simulink model "single_phase_grid_inverter"  (R2022b)
settings: Solver=FixedStepDiscrete  StartTime=0.0  StopTime=1.2  FixedStep=1e-6  RelTol=1e-3
libraries: spsSeriesRLCBranchLib x10, spsCurrentMeasurementLib x7, spsMosfetLib x6, spsVoltageMeasurementLib x6, spsFourierLib x4, spsRMSLib x4, spsIdealSwitchLib x2, spsMeanLib x2, simulink x2, spsDCVoltageSourceLib x1, spspowerguiLib x1, spsControlledVoltageSourceLib x1
settings Model: Creator=XIAO  LastModifiedBy=XIAO
settings SolverCC: AutoInsertRateTranBlk=on
settings DataIOCC: ReturnWorkspaceOutputs=off

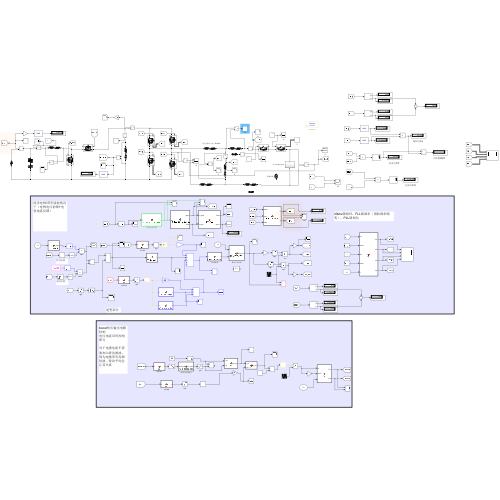
[thumbnail: Simulink's stored preview of the top-level diagram]
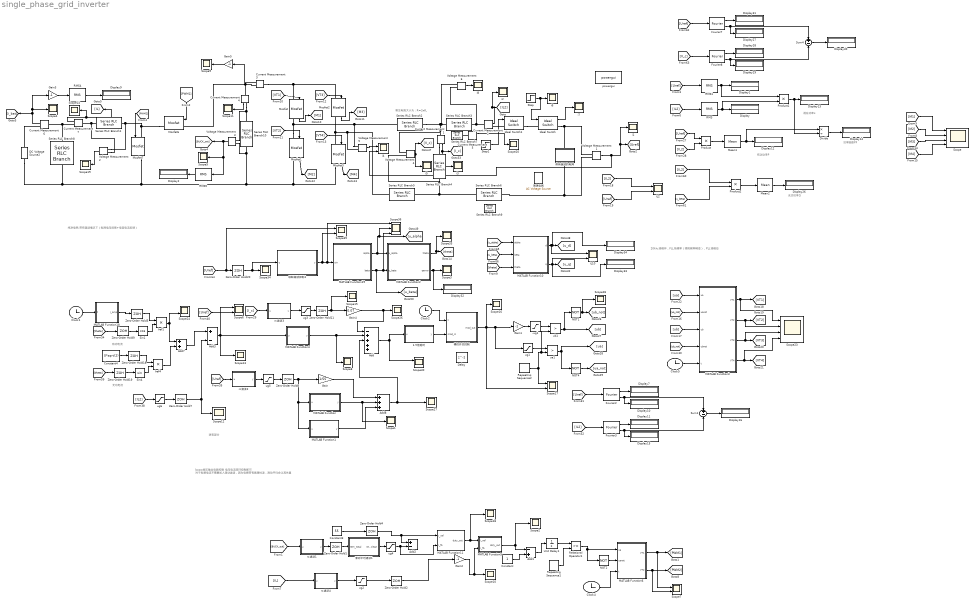
== system single_phase_grid_inverter ==
  note: 视在功率s
  note: 寄生电阻大小为：R=2πfL
  note: 功率因数PF
  note: 无功功率Q
  note: 有功电流
  note: 无功电流
  note: 纯净电网/带有谐波情况下（电网电压前馈+电容电流反馈）
  note: 有功功率P
  note: 逆变部分
  note: 20khz锁相环，FLL锁频率（预防频率畸变），PLL锁相位
  note: boost恒压输出电路控制
      | 电压电流双环控制即可
      |
      | 对于电感电流不需要加入滑动滤波，因为电感带有高频纹波，滑动平均会让其失真
  -ug1 : Saturate  UpperLimit=0.95  LowerLimit=-0.95
  1.5倍延时 : MATLAB Function  TreatAsAtomicUnit=on
  Add : Sum  Inputs=-++++
  Add1 : Sum  Inputs=-+
  Add2 : Sum  Inputs=+-
  Add3 : Sum  Inputs=+-
  Add7 : Sum
  Add8 : Sum  Inputs=+++
  Clock{1..2,4..5} (4 alike) : Clock
  Constant : Constant
  Constant3 : Constant  Value=55
  Constant4 : Constant  Value=0*sqrt(2)
  Current Measurement{1..7} (7 alike) : spsCurrentMeasurementLib/Current Measurement  PhasorSimulation=off  OutputType=Complex  PSBequivalent=0
  DC Voltage Source2 : spsDCVoltageSourceLib/DC Voltage Source  Amplitude=24  Measurements=None
  Delay : Delay  DelayLength=1  SampleTime=5e-5
  Display{,1..2,7,9..16,26..34} (21 alike) : Display
  Divide : Product  Inputs=*/
  Fourier{2..3,7..8} (4 alike) : spsFourierLib/Fourier  Freq=50  n=1  InInit=[0, 0]  Ts=1e-6
  Gain : Gain  Gain=1/55
  Gain{1..3,5} (4 alike) : Gain  Gain=-1
  Gain4 : Gain  Gain=0.07
  Ideal Switch : spsIdealSwitchLib/Ideal Switch  Ron=0.001  Lon=0  IC=0  Rs=1e5  Cs=inf  Measurements=on
  Ideal Switch1 : spsIdealSwitchLib/Ideal Switch  Ron=0.001  Lon=0  IC=0  Rs=1e5  Cs=inf  Measurements=on
  Iref1 : Product
  Iref4 : Product
  MATLAB Function : MATLAB Function  TreatAsAtomicUnit=on
  MATLAB Function1 : MATLAB Function  TreatAsAtomicUnit=on
  MATLAB Function10 : MATLAB Function  TreatAsAtomicUnit=on
  MATLAB Function11 : MATLAB Function  TreatAsAtomicUnit=on
  MATLAB Function18 : MATLAB Function  TreatAsAtomicUnit=on
  MATLAB Function19 : MATLAB Function  TreatAsAtomicUnit=on
  MATLAB Function2 : MATLAB Function  TreatAsAtomicUnit=on
  MATLAB Function3 : MATLAB Function  TreatAsAtomicUnit=on
  MATLAB Function4 : MATLAB Function  TreatAsAtomicUnit=on
  MATLAB Function5 : MATLAB Function  TreatAsAtomicUnit=on
  MATLAB Function6 : MATLAB Function  TreatAsAtomicUnit=on
  Mean1 : spsMeanLib/Mean  Freq=50  Vinit=0  Ts=5e-5
  Mean2 : spsMeanLib/Mean  Freq=50  Vinit=0  Ts=5e-5
  Mosfet{,1..3,6..7} (6 alike) : spsMosfetLib/Mosfet  Ron=0.1  Lon=0  Rd=0.01  Vfd=0  IC=0  Rs=1e5  Cs=inf  Measurements=on
  NOT1 : Logic  Operator=NOT  IconShape=distinctive  AllPortsSameDT=off  OutDataTypeStr=boolean
  NOT2 : Logic  Operator=NOT  IconShape=distinctive  AllPortsSameDT=off  OutDataTypeStr=boolean
  NOT4 : Logic  Operator=NOT  IconShape=distinctive  AllPortsSameDT=off  OutDataTypeStr=boolean
  Product : Product
  Product1 : Product
  Product2 : Product
  RMS : spsRMSLib/RMS  TrueRMS=on  Freq=50  RMSInit=24  Ts=1e-6
  RMS1 : spsRMSLib/RMS  TrueRMS=on  Freq=50  RMSInit=24  Ts=1e-6
  RMS4 : spsRMSLib/RMS  TrueRMS=on  Freq=50  RMSInit=120  Ts=1e-6
  RMS5 : spsRMSLib/RMS  TrueRMS=on  Freq=50  RMSInit=120  Ts=1e-6
  Relational Operator1 : RelationalOperator  OutDataTypeStr=boolean  RndMeth=Simplest  InputSameDT=off
  Repeating Sequence1 : simulink/Sources/Repeating Sequence  rep_seq_t=[0 0.00005 0.0001]  rep_seq_y=[0 1 0]
  Repeating Sequence2 : simulink/Sources/Repeating Sequence  rep_seq_t=[0, 5e-5, 1e-4]  rep_seq_y=[-1, 1, -1]
  Scope : Scope  NumInputPorts=4
  Scope{1..5,8..16,18..20,26..28,33..34} (22 alike) : Scope
  Scope{6..7,17,24,30,35} (6 alike) : Scope  NumInputPorts=2
  Scope23 : Scope  NumInputPorts=4
  Scope36 : Scope  NumInputPorts=3
  Series RLC Branch1 : spsSeriesRLCBranchLib/Series RLC Branch  LConnTagsString=__new0  RConnTagsString=__new0  BranchType=RL  Resistance=0.1  Inductance=2.5e-3  SetiL0=off  InitialCurrent=0  Capacitance=1e-6  Setx0=off  InitialVoltage=0  Measurements=None
  Series RLC Branch10 : spsSeriesRLCBranchLib/Series RLC Branch  LConnTagsString=__new0  RConnTagsString=__new0  BranchType=RC  Resistance=0.01  Inductance=0  SetiL0=off  InitialCurrent=0  Capacitance=1880e-6  Setx0=off  InitialVoltage=0  Measurements=None
  Series RLC Branch2 : spsSeriesRLCBranchLib/Series RLC Branch  LConnTagsString=__new0  RConnTagsString=__new0  BranchType=RL  Resistance=0.1  Inductance=0.0015  SetiL0=off  InitialCurrent=0  Capacitance=220e-6  Setx0=off  InitialVoltage=0  Measurements=None
  Series RLC Branch3 : spsSeriesRLCBranchLib/Series RLC Branch  LConnTagsString=__new0  RConnTagsString=__new0  BranchType=RL  Resistance=0.1  Inductance=0.00012  SetiL0=off  InitialCurrent=0  Capacitance=220e-6  Setx0=off  InitialVoltage=0  Measurements=None
  Series RLC Branch4 : spsSeriesRLCBranchLib/Series RLC Branch  LConnTagsString=__new0  RConnTagsString=__new0  BranchType=RC  Resistance=0.1  Inductance=0  SetiL0=off  InitialCurrent=0  Capacitance=10e-6  Setx0=off  InitialVoltage=0  Measurements=None
  Series RLC Branch5 : spsSeriesRLCBranchLib/Series RLC Branch  LConnTagsString=__new0  RConnTagsString=__new0  BranchType=RL  Resistance=0.1  Inductance=0.0015  SetiL0=off  InitialCurrent=0  Capacitance=220e-6  Setx0=off  InitialVoltage=0  Measurements=None
  Series RLC Branch6 : spsSeriesRLCBranchLib/Series RLC Branch  LConnTagsString=__new0  RConnTagsString=__new0  BranchType=RL  Resistance=0.1  Inductance=0.00012  SetiL0=off  InitialCurrent=0  Capacitance=220e-6  Setx0=off  InitialVoltage=0  Measurements=None
  Series RLC Branch7 : spsSeriesRLCBranchLib/Series RLC Branch  LConnTagsString=__new0  RConnTagsString=__new0  BranchType=RC  Resistance=10  Inductance=0.0000001  SetiL0=off  InitialCurrent=0  Capacitance=1e-7  Setx0=off  InitialVoltage=0  Measurements=None
  Series RLC Branch8 : spsSeriesRLCBranchLib/Series RLC Branch  LConnTagsString=__new0  RConnTagsString=__new0  BranchType=RC  Resistance=0.1  Inductance=1e-3  SetiL0=off  InitialCurrent=0  Capacitance=940e-6  Setx0=off  InitialVoltage=0  Measurements=None
  Series RLC Branch9 : spsSeriesRLCBranchLib/Series RLC Branch  LConnTagsString=__new0  RConnTagsString=__new0  BranchType=RC  Resistance=10  Inductance=0.0000001  SetiL0=off  InitialCurrent=0  Capacitance=1e-7  Setx0=off  InitialVoltage=0  Measurements=None
  Sin1 : Trigonometry  Operator=cos
  Sin4 : Trigonometry
  Step : Step  Time=0.26  SampleTime=1e-6
  Step1 : Step  Before=1  After=0  SampleTime=1e-6
  Sum1 : Sum  Inputs=+-
  Sum4 : Sum  Inputs=+-
  Unit Delay1 : UnitDelay  SampleTime=5e-5  HasFrameUpgradeWarning=on
  Voltage Measurement{1..6} (6 alike) : spsVoltageMeasurementLib/Voltage Measurement  PhasorSimulation=off  OutputType=Complex  PSBequivalent=0
  Zero-Order Hold{1..2,4..5,7..9,11,18..20} (11 alike) : ZeroOrderHold  SampleTime=5e-5
  i{1..3,5..8} (7 alike) : Scope
  i4 : Scope  NumInputPorts=2
  iL10 : Scope  NumInputPorts=2
  iL2 : Scope  NumInputPorts=2
  powergui : spspowerguiLib/powergui  Priority=1  SimulationMode=Discrete  SampleTime=1e-6  frequency=60  Iterations=50  frequencyindice=0  Pbase=100e6  ErrMax=1e-4  UnitsV=kV  UnitsW=MW  buscounter=0  FunctionMessages=off  echomessages=off  EnableUseOfTLC=off  CurrentSourceSwitches=off  DisableSnubberDevices=off  DisableRonSwitches=off  DisableVfSwitches=off  DisplayEquations=off  AutomaticDiscreteSolvers=off  SolverType=Tustin/Backward Euler (TBE)  Interpol=off  ExternalGateDelay=off  methode=off  Ts=100  x0status=blocks  SPID=on  SwTol=0  HookPort=off  NonlinearTolerance=1e-4  nMaxIteration=100  ContinueOnMaxIteration=off  RestoreLinks=warning  ResistiveCurrentMeasurement=off  Frange=[0:2:500]  Ylog=off  Xlog=on  ShowGrid=off  save=off  variable=ZData  structure=0  ZoomFFT=off  StartTime=0.0  cycles=1  DisplayStyle=1  fundamental=60  FreqAxis=off  MaxFrequency=1000  frequencyindicesteady=1  RmsSteady=1  display=off
  rc滤波1 : MATLAB Function  TreatAsAtomicUnit=on
  rc滤波2 : MATLAB Function  TreatAsAtomicUnit=on
  rc滤波3 : MATLAB Function  TreatAsAtomicUnit=on
  rc滤波4 : MATLAB Function  TreatAsAtomicUnit=on
  ua1 : RelationalOperator  Operator=>  OutDataTypeStr=boolean  RndMeth=Simplest  InputSameDT=off
  ub1 : RelationalOperator  Operator=>  OutDataTypeStr=boolean  RndMeth=Simplest  InputSameDT=off
  ug1 : Saturate  UpperLimit=0.95  LowerLimit=-0.95
  ug2 : Saturate  UpperLimit=10  LowerLimit=-10
  ug3 : Saturate  UpperLimit=5  LowerLimit=-5
  ug4 : Saturate  UpperLimit=60  LowerLimit=-60
  ug5 : Saturate  UpperLimit=5  LowerLimit=-5
  ug6 : Saturate  UpperLimit=10  LowerLimit=-10
  带有谐波的电网 : Subsystem
  模仿开关控制 : MATLAB Function  TreatAsAtomicUnit=on
  滑动平均滤波1 : MATLAB Function  TreatAsAtomicUnit=on
  理想电网 : spsACVoltageSourceLib/AC Voltage Source  Amplitude=24*1.414  Phase=0  Frequency=50  SampleTime=0  Measurements=None  BusType=swing  Pref=10e3  Qref=0  Qmin=-inf  Qmax=+inf
  级联谐波抑制4 : MATLAB Function  TreatAsAtomicUnit=on
  wires:
  [theta] -> Zero-Order Hold9/1
  [M2] -> Scope/2
  Fourier2/2 -> Display10/1, Sum1/1
  [VT1] -> Mosfet/1
  NOT1/1 -> Scope28/1, [ub_not]
  ub1/1 -> [ub], NOT1/1
  [M3] -> Scope/3
  Sin1/1 -> Iref1/2
  Fourier3/1 -> Display11/1
  Mean1/1 -> Divide/1, Display12/1
  [VT3] -> Mosfet2/1
  [IL2] -> Product/2
  [Uref] -> Product/1
  Product/1 -> Mean1/1
  [Uref] -> RMS1/1
  [IL2] -> RMS/1
  [VT4] -> Mosfet3/1
  [M1] -> Scope/1
  RMS/1 -> Product1/2, Display/1
  Sum1/1 -> Display16/1
  Add8/1 -> Add/3, Scope27/1
  模仿开关控制/1(mod_out) -> Scope16/1, Gain1/1, ug1/1, Scope17/2
  Iref4/1 -> Add7/2
  Fourier7/1 -> Display31/1
  1.5倍延时/1(y) -> 模仿开关控制/2(mod_in)
  Fourier8/2 -> Sum4/2, Display29/1
  MATLAB Function18/1(I_amp) -> Zero-Order Hold5/1
  Add/1 -> 1.5倍延时/1(u), Scope30/1
  Mean2/1 -> Display26/1
  Repeating Sequence2/1 -> ub1/2, ua1/2, Scope17/1
  [IL2] -> Product2/1
  Fourier8/1 -> Display28/1
  Zero-Order Hold9/1 -> Sin1/1
  Fourier2/1 -> Display7/1
  Gain4/1 -> Scope26/1, Add/1
  Zero-Order Hold7/1 -> Add3/2, Scope12/1
  Clock2/1 -> 模仿开关控制/1(t)
  MATLAB Function4/1(y) -> Add/2, Scope8/1
  [V_c] -> Fourier8/1
  Sum4/1 -> Display30/1
  Fourier7/2 -> Display27/1, Sum4/1
  [Uref] -> Fourier2/1
  Gain1/1 -> -ug1/1
  [Uref] -> Fourier7/1
  -ug1/1 -> ub1/1
  Gain/1 -> Add8/1
  Fourier3/2 -> Sum1/2, Display15/1
  Clock1/1 -> MATLAB Function18/1(t)
  Ideal Switch/1 -> i7/1
  Step/1 -> Ideal Switch/1, i6/1
  [I_c] -> rc滤波3/1(u)
  [theta] -> Zero-Order Hold19/1
  Product1/1 -> Divide/2, Display13/1
  Sin4/1 -> Iref4/2
  Current Measurement2/1 -> [IL2], i2/1
  Add3/1 -> Scope6/1, MATLAB Function4/1(u), Scope13/1
  [IL2] -> Fourier3/1
  Zero-Order Hold18/1 -> Iref4/1
  Product2/1 -> Mean2/1
  Zero-Order Hold19/1 -> Sin4/1
  [Uref] -> iL2/2
  RMS1/1 -> Product1/1, Display1/1
  MATLAB Function/1(y) -> Scope1/1, Add8/2
  Constant4/1 -> Zero-Order Hold18/1
  NOT4/1 -> [ua_not]
  Zero-Order Hold5/1 -> Iref1/1
  Mosfet/1 -> [M1]
  [IL2] -> ug6/1
  ug1/1 -> ua1/1
  Zero-Order Hold8/1 -> MATLAB Function1/1(u), MATLAB Function/1(u), Gain/1
  [Uref] -> rc滤波2/1(u)
  Current Measurement1/1 -> [I_c], i3/1
  Mosfet1/1 -> [M2]
  [u_beta] -> Product2/2
  Voltage Measurement4/1 -> i5/1, [V_c]
  [VT2] -> Mosfet1/1
  Mosfet3/1 -> [M4]
  ua1/1 -> [ua], NOT4/1
  Voltage Measurement1/1 -> i4/2, i1/1, [Uref]
  [M4] -> Scope/4
  [IL2] -> iL2/1
  Divide/1 -> Display14/1
  Add7/1 -> Add3/1
  Iref1/1 -> Add7/1, Scope24/2
  Mosfet2/1 -> [M3]
  [Uref] -> Scope6/2
  Zero-Order Hold2/1 -> Gain2/1
  MATLAB Function11/1(duty_out) -> Scope18/1, MATLAB Function5/1(I_ref)
  Repeating Sequence1/1 -> Relational Operator1/2
  Gain2/1 -> Scope10/1, MATLAB Function5/2(I_fb)
  Zero-Order Hold1/1 -> 滑动平均滤波1/1(IGm_total)
  Unit Delay1/1 -> Relational Operator1/1
  [BUCK_out] -> rc滤波1/1(u)
  Relational Operator1/1 -> NOT2/1, MATLAB Function6/1(ua)
  RMS4/1 -> Display9/1
  Voltage Measurement3/1 -> RMS5/1, Scope5/1, [BUCK_out]
  [PWM1] -> Mosfet6/1
  RMS5/1 -> Display2/1
  Current Measurement6/1 -> [i_bat], Scope4/1, Gain3/1
  [PWM2] -> Mosfet7/1
  Gain3/1 -> RMS4/1
  Current Measurement3/1 -> Gain5/1
  Gain5/1 -> Scope9/1
  Current Measurement4/1 -> Scope11/1
  Current Measurement7/1 -> Scope14/1, [IL]
  MATLAB Function2/2(qerror) -> Scope3/1, Display32/1
  MATLAB Function19/1(alpha) -> Scope36/2, [u_alpha], MATLAB Function2/1(u_alpha)
  MATLAB Function19/2(beta) -> Scope36/3, MATLAB Function2/2(u_beta), [u_beta]
  [u_alpha] -> MATLAB Function10/1(alpha)
  Zero-Order Hold20/1 -> 级联谐波抑制4/1(u), Scope34/1
  MATLAB Function2/1(theta) -> Scope33/1, [theta]
  级联谐波抑制4/1(y) -> Scope35/2, Scope36/1, MATLAB Function19/1(uin)
  [theta] -> MATLAB Function10/3(theta)
  MATLAB Function10/2(q) -> Display33/1, [u_q], iL10/2
  [Uref] -> Scope35/1, Zero-Order Hold20/1
  MATLAB Function10/1(d) -> iL10/1, Display34/1, [u_d]
  [u_beta] -> MATLAB Function10/2(beta)
  Zero-Order Hold11/1 -> Scope15/1, Gain4/1
  Constant3/1 -> Zero-Order Hold4/1
  Zero-Order Hold4/1 -> MATLAB Function11/1(I_ref), Add2/1
  [IL] -> rc滤波4/1(u)
  ug2/1 -> Zero-Order Hold2/1
  MATLAB Function5/1(duty_out) -> Add1/1, Scope2/1
  ug3/1 -> Zero-Order Hold11/1
  ug4/1 -> MATLAB Function11/2(I_fb), Add2/2
  ug5/1 -> Zero-Order Hold8/1
  MATLAB Function1/1(y) -> Add8/3
  Voltage Measurement2/1 -> Scope19/1
  Clock5/1 -> MATLAB Function3/5(t)
  MATLAB Function3/1(VT1) -> Scope23/1, [VT1]
  [ub] -> MATLAB Function3/3(ub)
  MATLAB Function3/2(VT2) -> Scope23/2, [VT2]
  [ua] -> MATLAB Function3/1(ua)
  MATLAB Function3/3(VT3) -> Scope23/3, [VT3]
  MATLAB Function3/4(VT4) -> Scope23/4, [VT4]
  [ub_not] -> MATLAB Function3/4(ubnot)
  [ua_not] -> MATLAB Function3/2(uanot)
  ug6/1 -> Zero-Order Hold7/1
  Step1/1 -> Ideal Switch1/1
  MATLAB Function6/1(VT1) -> [PWM1], Scope7/1
  NOT2/1 -> MATLAB Function6/2(uanot)
  Clock4/1 -> MATLAB Function6/3(t)
  MATLAB Function6/2(VT2) -> [PWM2], Scope7/2
  Constant/1 -> Add1/2
  Add1/1 -> Unit Delay1/1
  Voltage Measurement5/1 -> i4/1
  rc滤波1/1(y) -> Zero-Order Hold1/1
  rc滤波4/1(y) -> ug2/1
  滑动平均滤波1/1(IGm_clean) -> ug4/1
  rc滤波2/1(y) -> ug5/1
  rc滤波3/1(y) -> ug3/1
  Voltage Measurement6/1 -> i8/1
  Current Measurement5/1 -> Scope20/1
  connections:
  Ideal Switch/RConn1 -- Voltage Measurement1/LConn1 -- 带有谐波的电网/RConn1
  Mosfet2/RConn1 -- Voltage Measurement5/LConn2 -- Series RLC Branch5/RConn1 -- Mosfet3/LConn1
  Voltage Measurement3/LConn2 -- Series RLC Branch10/RConn1 -- Mosfet7/RConn1 -- Series RLC Branch8/RConn1 -- DC Voltage Source2/LConn1 -- Mosfet1/RConn1 -- Mosfet3/RConn1
  Mosfet1/LConn1 -- Voltage Measurement5/LConn1 -- Series RLC Branch2/RConn1 -- Mosfet/RConn1
  Series RLC Branch2/LConn1 -- Current Measurement1/LConn1 -- Voltage Measurement4/LConn1 -- Series RLC Branch3/RConn1 -- Voltage Measurement6/LConn1
  Current Measurement2/LConn1 -- Voltage Measurement6/LConn2 -- Series RLC Branch3/LConn1
  Current Measurement1/RConn1 -- Series RLC Branch4/LConn1
  Series RLC Branch8/LConn1 -- Current Measurement7/RConn1 -- Current Measurement6/LConn1
  Mosfet6/RConn1 -- Voltage Measurement2/LConn1 -- Series RLC Branch1/LConn1 -- Mosfet7/LConn1
  Current Measurement3/RConn1 -- Current Measurement4/LConn1 -- Mosfet6/LConn1
  Series RLC Branch1/RConn1 -- Voltage Measurement2/LConn2 -- Current Measurement7/LConn1
  Current Measurement6/RConn1 -- DC Voltage Source2/RConn1
  Series RLC Branch4/RConn1 -- Voltage Measurement4/LConn2 -- Series RLC Branch6/RConn1 -- Series RLC Branch5/LConn1
  Voltage Measurement1/LConn2 -- 带有谐波的电网/LConn1 -- Series RLC Branch6/LConn1
  Mosfet2/LConn1 -- Current Measurement3/LConn1 -- Mosfet/LConn1
  Voltage Measurement3/LConn1 -- Series RLC Branch10/LConn1 -- Current Measurement4/RConn1
  Ideal Switch1/LConn1 -- Current Measurement2/RConn1
  Ideal Switch1/RConn1 -- Ideal Switch/LConn1
  Current Measurement5/LConn1 -- Series RLC Branch7/LConn1

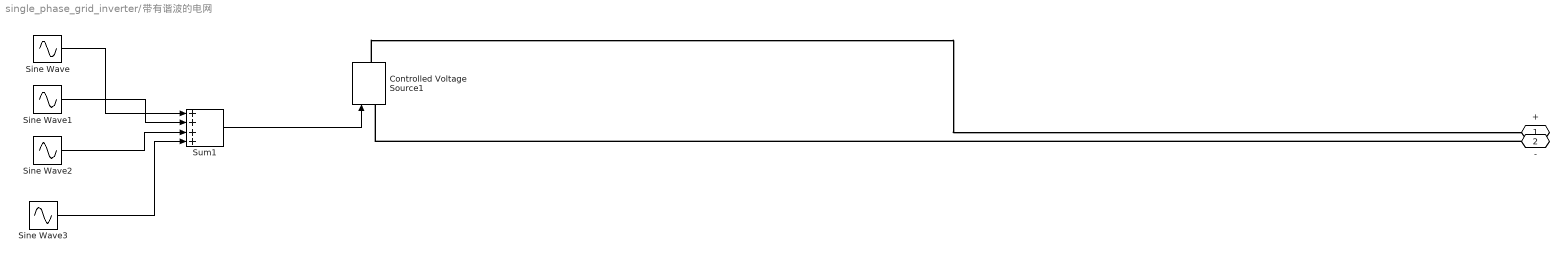
== system single_phase_grid_inverter/带有谐波的电网 ==
  Controlled Voltage Source1 : spsControlledVoltageSourceLib/Controlled Voltage Source  Initialize=off  Source_Type=AC  Amplitude=0  Phase=0  Frequency=0  Measurements=Voltage
  Sine Wave : Sin  Amplitude=32*sqrt(2)  Frequency=100*pi  SampleTime=0
  Sine Wave1 : Sin  Amplitude=0.04*32*sqrt(2)  Frequency=300*pi  SampleTime=0
  Sine Wave2 : Sin  Amplitude=0.03*32*sqrt(2)  Frequency=500*pi  SampleTime=0
  Sine Wave3 : Sin  Amplitude=0.02*32*sqrt(2)  Frequency=700*pi  SampleTime=0
  Sum1 : Sum  Inputs=++++
  + : PMIOPort  Side=Right
  - : PMIOPort  Port=2  Side=Left
  wires:
  Sum1/1 -> Controlled Voltage Source1/1
  Sine Wave1/1 -> Sum1/2
  Sine Wave/1 -> Sum1/1
  Sine Wave3/1 -> Sum1/4
  Sine Wave2/1 -> Sum1/3
  connections:
  -/RConn1 -- Controlled Voltage Source1/LConn1
  Controlled Voltage Source1/RConn1 -- +/RConn1

== matlab function single_phase_grid_inverter/MATLAB Function11 ==
  data: I_ref input; duty_out output; I_fb input
function duty_out = fcn(I_ref, I_fb)
%#codegen
% 同步Boost电流环PI控制器（带钳位抗饱和）
% 适配：20kHz采样、±5A电流传感器、占空比0.1~0.9安全范围
% 输入：
%   I_ref: 电压环输出的电流给定（对应你模型里电压环PI的输出）
%   I_fb: 电流反馈（对应你模型里经过-1增益后的IL信号）
% 输出：
%   duty_out: 最终占空比，直接接你模型里的1/z延迟模块

% 持久化变量：保存积分器状态，每个控制周期保留数值
persistent integral_val;
% 初始化：仅仿真启动的第一个控制周期执行1次
if isempty(integral_val)
    integral_val = 0;
end

% ==================== 1. 控制参数（和你原PI模块参数完全一致，可直接修改）====================
Kp = 0.5;       % 比例增益，和你原设置一致
Ki = 10;         % 积分增益，和你原设置一致
Ts = 5e-5;       % 20kHz控制周期，固定不变
% ==================== 2. 物理极限设置（核心抗饱和阈值）====================
DUTY_MAX = 100;  % 占空比上限，避免上下管直通
DUTY_MIN = -100;  % 占空比下限，杜绝轻载反向电流
I_SAT_LIMIT = 60; % 电流传感器饱和阈值，接近±5A量程提前触发保护

% ==================== 3. 误差计算 ====================
err = I_ref - I_fb;

% ==================== 4. 比例项输出 ====================
prop_out = Kp * err;

% ==================== 5. 核心抗饱和逻辑 ====================
% 5.1 积分项预计算
integral_inc = Ki * Ts * err;
integral_pre = integral_val + integral_inc;
% 5.2 预计算不饱和的PI输出
duty_pre = prop_out + integral_pre;

% 5.3 钳位抗饱和规则：
% 仅当输出在线性区、且电流未达到传感器饱和阈值时，才允许积分累加
% 同时加入反向积分放行规则，避免积分锁死
is_duty_linear = (duty_pre < DUTY_MAX) && (duty_pre > DUTY_MIN);
is_current_unsat = (abs(I_fb) < I_SAT_LIMIT);
is_integral_allow = is_duty_linear && is_current_unsat;
is_reverse_integral = (err > 0 && integral_pre < 0) || (err < 0 && integral_pre > 0);

if is_integral_allow || is_reverse_integral
    integral_val = integral_pre;
end

% ==================== 6. 最终占空比计算 + 硬限幅兜底 ====================
duty_out = prop_out + integral_val;
duty_out = min(max(duty_out, DUTY_MIN), DUTY_MAX);

== matlab function single_phase_grid_inverter/滑动平均滤波1 ==
  data: IGm_total input; IGm_clean output
function IGm_clean = Notch_100Hz_IGm(IGm_total)
    % 【动态窗口滑动平均滤波】专门消除100Hz纹波
    % 采样频率：20kHz，窗口长度：200点（20kHz/100Hz=200）
    % 核心改进：启动前200个点使用动态窗口，完全消除零值误差
    % 输入：IGm_total - 原始带纹波的电流信号
    % 输出：IGm_clean - 滤波后的平滑电流信号
    
    % 持久变量：仅在第一次调用时初始化，后续调用保留值
    persistent buffer   % 环形数据缓冲区
    persistent index    % 缓冲区当前写入索引
    persistent sum_buf  % 窗口内数据累加和（优化计算，避免循环求和）
    persistent sample_count % 已采样总点数（用于动态窗口判断）
    
    N = 200; % 固定窗口长度：100Hz纹波的精确零点
    
    % ====================== 初始化（仅第一次运行执行） ======================
    if isempty(buffer)
        buffer = zeros(1, N);  % 初始化环形缓冲区为全0
        index = 0;             % 索引从0开始
        sum_buf = 0;           % 累加和初始化为0
        sample_count = 0;      % 采样计数初始化为0
    end
    
    % ====================== 更新索引和计数 ======================
    sample_count = sample_count + 1; % 总采样数+1
    index = index + 1;
    if index > N
        index = 1; % 索引越界时回到起点，实现环形结构
    end
    
    % ====================== 核心滤波逻辑 ======================
    if sample_count <= N
        % ---------------------- 阶段1：动态窗口（前200个点） ----------------------
        % 不除以固定的200，而是除以当前已采样的点数
        % 第1个点：输出 = 第1个点 / 1
        % 第10个点：输出 = 前10个点和 / 10
        % ...
        % 第200个点：输出 = 前200个点和 / 200
        sum_buf = sum_buf + IGm_total;
        buffer(index) = IGm_total;
        IGm_clean = sum_buf / sample_count;
    else
        % ---------------------- 阶段2：标准滑动平均（200个点之后） ----------------------
        % 窗口已满，进入标准滑动模式
        % 减去最旧的采样值，加上最新的采样值
        sum_buf = sum_buf - buffer(index) + IGm_total;
        buffer(index) = IGm_total;
        IGm_clean = sum_buf / N;
    end
end

% 
% function IGm_clean = Notch_100Hz_IGm(IGm_total)
%     % 【标准固定窗口滑动平均滤波】专门消除100Hz纹波
%     % 采样频率：20kHz，窗口长度：200点（20kHz/100Hz=200）
%     % 输入：IGm_total - 原始带纹波的电流信号
%     % 输出：IGm_clean - 滤波后的平滑电流信号
%     
%     % 持久变量：仅在第一次调用时初始化，后续调用保留值
%     persistent buffer   % 环形数据缓冲区
%     persistent index    % 缓冲区当前写入索引
%     persistent sum_buf  % 窗口内数据累加和（优化计算，避免循环求和）
%     
%     N = 200; % 固定窗口长度：100Hz纹波的精确零点
%     
%     % ====================== 初始化（仅第一次运行执行） ======================
%     if isempty(buffer)
%         buffer = zeros(1, N);  % 初始化环形缓冲区为全0
%         index = 0;             % 索引从0开始
%         sum_buf = 0;           % 累加和初始化为0
%     end
%     
%     % ====================== 更新环形缓冲区索引 ======================
%     index = index + 1;
%     if index > N
%         index = 1; % 索引越界时回到起点，实现环形结构
%     end
%     
%     % ====================== 核心滤波逻辑（固定窗口） ======================
%     % 减去最旧的采样值，加上最新的采样值
%     sum_buf = sum_buf - buffer(index) + IGm_total;
%     
%     % 将最新的采样值存入缓冲区
%     buffer(index) = IGm_total;
%     
%     % 计算平均值（滤波输出）
%     IGm_clean = sum_buf / N;
% end

== matlab function single_phase_grid_inverter/MATLAB Function18 ==
  data: t input; I_amp output
function I_amp = current_amp_step(t)
% 功能：0.25s前输出0；0.25s~0.6s线性增长到2*sqrt(2)；0.6s后保持最大值不变
% 输入：t - 时间
% 输出：I_amp - 输出电流幅值

persistent I_target t_start t_end;
if isempty(I_target)
    I_target = 2*sqrt(2);  % 目标峰值：2*根号2 ≈2.828
    t_start  = 0.25;       % 线性增长起始时间
    t_end    = 0.6;        % 线性增长结束时间
end

% 分段逻辑
if t < t_start
    % 0 ~ 0.25s：输出0
    I_amp = 0;
elseif t <= t_end
    % 0.25s ~ 0.6s：线性增长计算
    % 公式：当前值 = 目标值 × (当前时间-起始时间)/总增长时间
    I_amp = I_target * (t - t_start) / (t_end - t_start);
else
    % 大于0.6s：保持最大值不变
    I_amp = I_target;
end
end

== matlab function single_phase_grid_inverter/模仿开关控制 ==
  data: t input; mod_out output; mod_in input
function mod_out = gate_mod_signal(t, mod_in)
% 功能：0.25s前输出0，0.25s后输出原调制波mod_in
% 输入 t: 仿真时间 (Clock模块)
% 输入 mod_in: 原始调制波信号
% 输出 mod_out: 带使能的调制波信号

t_start = 0.25; % 合闸时间

if t < t_start
    mod_out = 0;          % 合闸前强制输出0
else
    mod_out = mod_in;      % 合闸后输出原调制波
end
end

== matlab function single_phase_grid_inverter/MATLAB Function10 ==
  data: alpha input; d output; beta input; theta input; q output
function [d, q] = Park_Transform(alpha, beta, theta)
% Park变换模块（直接输入SOGI-FLL的theta，无内部积分）
% 输入：
%   alpha - α轴分量（SOGI-FLL的U_prime）
%   beta  - β轴分量（SOGI-FLL的deltaU_prime）
%   theta - 瞬时相位（SOGI-FLL直接输出的theta）
% 输出：
%   d         - d轴（直轴）分量
%   q         - q轴（交轴）分量
%   cos_theta - 相位θ的余弦值（新增输出）
%   sin_theta - 相位θ的正弦值（新增输出）

%% 核心计算
cos_theta = cos(theta);  % 相位θ的余弦值
sin_theta = sin(theta);  % 相位θ的正弦值


% 修正后的 Park 变换公式（d轴对齐同相分量 beta）
d =  alpha * cos_theta + beta * sin_theta;
q = -alpha * sin_theta + beta * cos_theta;
end

== matlab function single_phase_grid_inverter/MATLAB Function1 ==
  data: u input; y output
function y = GridVoltageFeedforward_Deriv_Module(u)
%#codegen
% 电网电压全前馈二阶微分模块
% 新增：频率预畸变（Frequency Prewarping），修正双线性变换的频率畸变
% 输入u：电网电压采样值 vg
% 输出y：模块输出信号

%% ===================== 1. 系统参数定义 =====================
L1 = 1.5e-3;         % 逆变侧电感，H
C = 10e-6;           % 滤波电容，F
k_pwm = 55;          % PWM桥臂增益
Ts = 1/20000;        % 采样周期，s（20kHz）
f_cutoff = 1150;     % 二阶低通截止频率，Hz（数字域目标频率）
zeta = 0.707;        % 阻尼系数（Butterworth）

%% ===================== 2. 频率预畸变（核心新增） =====================
% 数字域目标角频率
omega_d = 2 * pi * f_cutoff;
% 频率预畸变公式：omega_prewarp = (2/Ts) * tan(omega_d * Ts / 2)
% 目的：让双线性变换后的数字滤波器截止频率精确等于目标f_cutoff
omega_s = (2 / Ts) * tan(omega_d * Ts / 2);

%% ===================== 3. 双线性变换系数计算（使用预畸变后的omega_s） =====================
a = 2 / Ts;  % 双线性变换核心系数
K = (L1 * C) / k_pwm;  % 模块基础比例系数

% 分子系数
num2 = K * (omega_s^2) * (a^2);
num1 = -2 * num2;
num0 = num2;

% 分母系数
den2 = a^2 + 2 * zeta * omega_s * a + omega_s^2;
den1 = -2 * a^2 + 2 * omega_s^2;
den0 = a^2 - 2 * zeta * omega_s * a + omega_s^2;

%% ===================== 4. 状态变量初始化 =====================
persistent u_prev1 u_prev2 y_prev1 y_prev2;
if isempty(u_prev1)
    u_prev1 = 0; % u(k-1)
    u_prev2 = 0; % u(k-2)
    y_prev1 = 0; % y(k-1)
    y_prev2 = 0; % y(k-2)
end

%% ===================== 5. 差分方程实现 =====================
num_part = num2 * u + num1 * u_prev1 + num0 * u_prev2;
den_part = den1 * y_prev1 + den0 * y_prev2;
y = (num_part - den_part) / den2;

%% ===================== 6. 更新状态变量 =====================
u_prev2 = u_prev1;
u_prev1 = u;
y_prev2 = y_prev1;
y_prev1 = y;

end

== matlab function single_phase_grid_inverter/MATLAB Function19 ==
  settings: updateMethod=DISCRETE
  data: uin input; alpha output; beta output
% function [alpha, beta] = SOGI_FLL_20kHz(uin)
% % 严格对应你的 m 文件：20kHz 双线性 PI-FLL
% % 输入：uin   单相电压
% % 输出：alpha 同相输出 uα = x2
% %      beta  正交输出 uβ = omega0*x3
% 
% %% 固定参数（和你的m文件完全一致）
% dt = 5e-5;
% K  = 1.414;
% K1 = 0.25;
% gamma_p =30;
% gamma_i =500;
% w_max = 2*pi*60;
% w_min = 2*pi*40;
% 
% %% 状态持久化
% persistent x1_prev x2_prev x3_prev omega0_prev U_prev integral_f first_run;
% if isempty(first_run)
%     x1_prev = 0;
%     x2_prev = 0;
%     x3_prev = 0;
%     omega0_prev = 2*pi*50;
%     U_prev = uin;
%     integral_f = 0;
%     first_run = false;
% end
% 
% %% 1. 当前输入
% U_curr = uin;
% omega0_prev_local = omega0_prev;
% 
% %% 2. 频率预畸变
% omega_pre = (2/dt) * tan(omega0_prev_local * dt / 2);
% 
% %% 3. 状态矩阵 A, B
% A_mat = [
%     -K1*omega_pre, -K1*omega_pre, 0;
%     -K*omega_pre,  -K*omega_pre,  -omega_pre^2;
%     0,              1,              0
% ];
% B_mat = [
%     K1*omega_pre;
%     K*omega_pre;
%     0
% ];
% 
% %% 4. 双线性变换
% I_mat = eye(3);
% M1 = I_mat - (dt/2)*A_mat;
% M2 = I_mat + (dt/2)*A_mat;
% U_avg = U_curr + U_prev;
% 
% x_prev_vec = [x1_prev; x2_prev; x3_prev];
% x_curr_vec = M1 \ (M2 * x_prev_vec + (dt/2)*B_mat * U_avg);
% 
% x1_curr = x_curr_vec(1);
% x2_curr = x_curr_vec(2);
% x3_curr = x_curr_vec(3);
% 
% %% 5. PI-FLL 频率环
% deltaU = U_curr - x1_curr - x2_curr;
% deltaU_prime_val = omega0_prev_local * x3_curr;
% epsilon_f = deltaU * deltaU_prime_val;
% 
% integral_f = integral_f + epsilon_f * dt;
% domega0dt = -gamma_p * epsilon_f - gamma_i * integral_f;
% omega0_curr = omega0_prev_local + dt * domega0dt;
% 
% % 频率限幅
% omega0_curr = max(min(omega0_curr, w_max), w_min);
% 
% %% 6. 输出 alpha beta
% alpha = x2_curr;
% beta  = omega0_curr * x3_curr;
% 
% %% 7. 更新状态
% x1_prev = x1_curr;
% x2_prev = x2_curr;
% x3_prev = x3_curr;
% omega0_prev = omega0_curr;
% U_prev = U_curr;
% 
% end

function [alpha, beta] = SOGI_FLL_20kHz_Optimized(uin)
% 优化版 SOGI-FLL (针对嵌入式提速)
% 输入：uin - 单相电压采样
% 输出：alpha - 同相分量, beta - 正交分量

%% 固定参数
dt = 5e-5;           % 50us
h  = dt / 2;         % 中间步长
K  = 1.41421356;     % sqrt(2)
K1 = 0.25;
gamma_p = 30;
gamma_i = 500;
w_max = 2 * pi * 60;
w_min = 2 * pi * 40;

%% 状态持久化
persistent x1_prev x2_prev x3_prev omega0_prev U_prev integral_f first_run;
if isempty(first_run)
    x1_prev = 0; x2_prev = 0; x3_prev = 0;
    omega0_prev = 2 * pi * 50;
    U_prev = uin;
    integral_f = 0;
    first_run = false;
end

%% 1. 频率近似 (提速核心 1)
% 原逻辑：omega_pre = (2/dt) * tan(omega0_prev * dt / 2)
% 近似逻辑：当 dt 很小时，tan(x) ≈ x，则 omega_pre ≈ omega0_prev
% 20kHz下，50Hz对应的角度约为 0.0078 rad，近似误差极小
omega_pre = omega0_prev; 
U_avg = uin + U_prev;

%% 2. 预计算常数与中间变量
w_h = omega_pre * h;
wp_sq_h = omega_pre * omega_pre * h;
h_K1w = h * K1 * omega_pre;
h_Kw  = h * K * omega_pre;

% 展开 M2 矩阵与向量乘法: R = M2 * x_prev + h * B * U_avg
% M2 = [1-hK1w, -hK1w, 0; -hKw, 1-hKw, -h*w^2; 0, h, 1]
r1 = (1 - h_K1w)*x1_prev - h_K1w*x2_prev + h_K1w*U_avg;
r2 = -h_Kw*x1_prev + (1 - h_Kw)*x2_prev - wp_sq_h*x3_prev + h_Kw*U_avg;
r3 = h*x2_prev + x3_prev;

%% 3. 代数解析解 (提速核心 2: 消除矩阵求逆)
% 求解 M1 * x_curr = R
% M1 矩阵元素：
% m11 = 1+hK1w; m12 = hK1w; 
% m21 = hKw;    m22 = 1+hKw;  m23 = h*w^2;
% m31 = 0;      m32 = -h;     m33 = 1;

% 利用稀疏性手动降元求解 2x2 方程组
% 步骤 A: x3 = r3 + h*x2
% 步骤 B: 代入第二行消去 x3
a = 1 + h_K1w;
b = h_K1w;
c = h_Kw;
d = 1 + h_Kw + h * wp_sq_h; % 合并项：m22 - m23*(-h)
e = r1;
f = r2 - wp_sq_h * r3;      % 合并项：r2 - m23*r3

% 克莱姆法则求解
det_inv = 1 / (a * d - b * c);
x1_curr = (e * d - b * f) * det_inv;
x2_curr = (a * f - c * e) * det_inv;
x3_curr = r3 + h * x2_curr;

%% 4. FLL 频率环 (保持原逻辑)
deltaU = uin - x1_curr - x2_curr;
epsilon_f = deltaU * (omega_pre * x3_curr);
integral_f = integral_f + epsilon_f * dt;
domega0dt = -gamma_p * epsilon_f - gamma_i * integral_f;
omega0_curr = omega_pre + dt * domega0dt;

% 频率限幅
if omega0_curr > w_max, omega0_curr = w_max; end
if omega0_curr < w_min, omega0_curr = w_min; end

%% 5. 输出与状态更新
alpha = x2_curr;
beta  = omega0_curr * x3_curr;

x1_prev = x1_curr;
x2_prev = x2_curr;
x3_prev = x3_curr;
omega0_prev = omega0_curr;
U_prev = uin;

end

== matlab function single_phase_grid_inverter/MATLAB Function2 ==
  data: u_alpha input; theta output; u_beta input; qerror output
function [theta, qerror] = SRF_PLL(u_alpha, u_beta)
% 同步旋转坐标系锁相环 SRF-PLL
% 【已修改为：纯自适应频率版本 → 和你主循环PLL完全一致】
% 输入：u_alpha, u_beta
% 输出：theta 锁相相位, qerror q分量（趋近0）

    %% ===================== 1. 固定参数 =====================
    Ts = 5e-5;               % 20kHz 采样步长（必须匹配）
    
    % PI参数（和你主循环一致）
    kp_pll = 200;
    ki_pll = 7000;

    %% ===================== 2. 持久变量 =====================
    persistent theta_prev
    persistent integral_pll
    
    if isempty(theta_prev)
        theta_prev = 0;
        integral_pll = 0;
    end

    %% ===================== 3. Park 变换 =====================
    cos_theta = cos(theta_prev);
    sin_theta = sin(theta_prev);
    
    u_d =  u_alpha * cos_theta + u_beta * sin_theta;
    u_q = -u_alpha * sin_theta + u_beta * cos_theta;
    
    qerror = u_q;  % q分量（锁相成功→0）

    %% ===================== 4. PI控制器（我的版本：直接输出ω） =====================
    integral_pll = integral_pll + qerror * Ts;          % 积分
    omega_pll    = kp_pll * qerror + ki_pll * integral_pll; % 直接输出角频率

    %% ===================== 5. 积分生成相位 =====================
    theta = theta_prev + omega_pll * Ts;

    %% ===================== 6. 相位归一化（±π） =====================
    if theta > pi
        theta = theta - 2*pi;
    elseif theta < -pi
        theta = theta + 2*pi;
    end

    %% ===================== 7. 更新状态 =====================
    theta_prev = theta;
end

== matlab function single_phase_grid_inverter/级联谐波抑制4 ==
  data: u input; y output
function y = Cascade_Notch_Filter(u)
% 级联陷波滤波器：滤除3/5/7次固定频率谐波（150/250/350Hz）
% 输入u：待滤波的标量信号
% 输出y：滤波后的标量信号
% 适配：20kHz采样率（Ts=5e-5），和你的控制环完全对齐

    persistent x3_1 x3_2 x5_1 x5_2 x7_1 x7_2 first_run
    persistent b3_0 b3_1 b3_2 a3_1 a3_2
    persistent b5_0 b5_1 b5_2 a5_1 a5_2
    persistent b7_0 b7_1 b7_2 a7_1 a7_2

    %% ===================== 1. 初始化：仅首次运行 =====================
    if isempty(first_run)
        % --- 固定参数 ---
        Fs = 2e4;          % 采样频率 20kHz
        Ts = 1/Fs;            % 采样周期 5e-5s
        wc = 10;              % 截止角频率 25 rad/s
        
        % 目标谐波频率
        w3 = 2*pi*150;  % 3次谐波 150Hz
        w5 = 2*pi*250;  % 5次谐波 250Hz
        w7 = 2*pi*350;  % 7次谐波 350Hz

        % --- Tustin变换预计算系数 ---
        k = 2/Ts;
        k2 = k*k;

        % --- 3次滤波器系数 ---
        [b3_0, b3_1, b3_2, a3_1, a3_2] = calc_coeff(w3, wc, k, k2);
        % --- 5次滤波器系数 ---
        [b5_0, b5_1, b5_2, a5_1, a5_2] = calc_coeff(w5, wc, k, k2);
        % --- 7次滤波器系数 ---
        [b7_0, b7_1, b7_2, a7_1, a7_2] = calc_coeff(w7, wc, k, k2);

        % --- 显式初始化状态变量为标量 ---
        x3_1 = 0; x3_2 = 0;
        x5_1 = 0; x5_2 = 0;
        x7_1 = 0; x7_2 = 0;
        
        first_run = 1;
    end

    %% ===================== 2. 级联滤波计算（显式差分方程） =====================
    % --- 第1级：3次谐波滤波 ---
    y3 = b3_0*u + x3_1;
    x3_1_next = b3_1*u - a3_1*y3 + x3_2;
    x3_2_next = b3_2*u - a3_2*y3;
    
    % --- 第2级：5次谐波滤波 ---
    y5 = b5_0*y3 + x5_1;
    x5_1_next = b5_1*y3 - a5_1*y5 + x5_2;
    x5_2_next = b5_2*y3 - a5_2*y5;
    
    % --- 第3级：7次谐波滤波 ---
    y7 = b7_0*y5 + x7_1;
    x7_1_next = b7_1*y5 - a7_1*y7 + x7_2;
    x7_2_next = b7_2*y5 - a7_2*y7;
    
    % --- 更新状态变量 ---
    x3_1 = x3_1_next; x3_2 = x3_2_next;
    x5_1 = x5_1_next; x5_2 = x5_2_next;
    x7_1 = x7_1_next; x7_2 = x7_2_next;
    
    % --- 最终输出 ---
    y = y7;

end

%% ===================== 局部函数：预计算滤波器系数 =====================
function [b0, b1, b2, a1, a2] = calc_coeff(wn, wc, k, k2)
    % 连续域：G(s) = (s^2 + wn^2) / (s^2 + 2*wc*s + wn^2)
    % Tustin离散化：s = k*(z-1)/(z+1)
    
    % 连续域系数
    num_b0 = 1; num_b1 = 0; num_b2 = wn^2;
    den_a0 = 1; den_a1 = 2*wc; den_a2 = wn^2;
    
    % 离散化计算
    B0 = num_b0*k2 + num_b1*k + num_b2;
    B1 = 2*num_b2 - 2*num_b0*k2;
    B2 = num_b0*k2 - num_b1*k + num_b2;
    
    A0 = den_a0*k2 + den_a1*k + den_a2;
    A1 = 2*den_a2 - 2*den_a0*k2;
    A2 = den_a0*k2 - den_a1*k + den_a2;
    
    % 归一化（a0=1）
    b0 = B0 / A0;
    b1 = B1 / A0;
    b2 = B2 / A0;
    a1 = A1 / A0;
    a2 = A2 / A0;
end

== matlab function single_phase_grid_inverter/MATLAB Function ==
  data: u input; y output
function y = CapCurrentDamping(u)
%#codegen
% 电容电流反馈有源阻尼环节
% 离散化方法：双线性变换法（Tustin），fs=20kHz
% 输入u：电容电压采样值
% 输出y：有源阻尼反馈信号

%% 固定参数（和你的系统匹配）
persistent u_prev  % 上一拍的输入值 u(k-1)
persistent y_prev  % 上一拍的输出值 y(k-1)
C = 10e-6;          % 滤波电容，F
Hi1 = 0.07;          % 反馈系数
Ts = 1/20000;        % 采样周期，s

%% 初始化状态变量
if isempty(u_prev)
    u_prev = 0;
    y_prev = 0;
end

%% 双线性变换法（Tustin）实现微分
% 连续域：G(s) = C*Hi1 * s
% 双线性变换：s = (2/Ts) * (z-1)/(z+1)
% 差分方程：y(k) = -y(k-1) + (2*C*Hi1/Ts) * (u(k) - u(k-1))
K_tustin = (2 * C * Hi1) / Ts;
y = -y_prev + K_tustin * (u - u_prev);

%% 更新状态变量
u_prev = u;
y_prev = y;
end



% function y = CapCurrentDamping_Improved(u)
% %#codegen
% % 电容电流反馈有源阻尼环节（改进版：微分 + 1kHz一阶低通）
% % 特点：绝对稳定，抑制开关噪声，和STM32 C代码逐行对应
% % 离散化方法：双线性变换法（Tustin）+ 频率预畸变，fs=20kHz
% % 输入u：电容电压采样值
% % 输出y：有源阻尼反馈信号
% 
% %% 持久化变量（保存状态和预计算系数）
% persistent u_prev  % 上一拍的输入值 u(k-1)
% persistent y_prev  % 上一拍的输出值 y(k-1)
% persistent b0 b1 a1 % 预计算的离散化系数
% 
% %% 固定参数（和你的系统匹配）
% C = 10e-6;          % 滤波电容，F
% Hi1 = 0.07;          % 反馈系数
% Ts = 1/20000;        % 采样周期，s
% f_cutoff = 1000;     % 【关键】低通截止频率 1kHz
% 
% %% 初始化：仅在第一次运行时执行
% if isempty(u_prev)
%     u_prev = 0;
%     y_prev = 0;
%     
%     % 1. 计算截止角频率
%     omega_c = 2.0 * pi * f_cutoff;
%     
%     % 2. 频率预畸变：让数字截止频率精准对应模拟截止频率
%     omega_s = (2.0 / Ts) * tan(omega_c * Ts / 2.0);
%     
%     % 3. 预计算差分方程系数 (和C代码完全一致)
%     a0 = 2.0 + omega_s * Ts;
%     
%     b0 = (2.0 * C * Hi1 * omega_s) / a0;
%     b1 = -b0;
%     a1 = (omega_s * Ts - 2.0) / a0;
% end
% 
% %% 核心差分方程（每一拍运行）
% % 公式：y(k) = b0*u(k) + b1*u(k-1) - a1*y(k-1)
% y = b0 * u + b1 * u_prev - a1 * y_prev;
% 
% 
% 
% %% 更新状态变量
% u_prev = u;
% y_prev = y;
% 
% end

== matlab function single_phase_grid_inverter/MATLAB Function6 ==
  data: ua input; VT1 output; uanot input; t input; VT2 output
function [VT1, VT2] = fcn(ua, uanot, t)
% 分段 PWM 输出控制
% t < 0.25s       → 全 0
% 0.25s ≤ t < 1s  → 正常输出
% t ≥ 1s          → 再次全 0

if t < 0.9
    VT1 = ua;
    VT2 = uanot;
else
    VT1 = false;
    VT2 = false;
end
   
end

== matlab function single_phase_grid_inverter/MATLAB Function5 ==
  data: I_ref input; duty_out output; I_fb input
function duty_out = fcn(I_ref, I_fb)
%#codegen
% 同步Boost电流环PI控制器（带钳位抗饱和）
% 适配：20kHz采样、±5A电流传感器、占空比0.1~0.9安全范围
% 输入：
%   I_ref: 电压环输出的电流给定（对应你模型里电压环PI的输出）
%   I_fb: 电流反馈（对应你模型里经过-1增益后的IL信号）
% 输出：
%   duty_out: 最终占空比，直接接你模型里的1/z延迟模块

% 持久化变量：保存积分器状态，每个控制周期保留数值
persistent integral_val;
% 初始化：仅仿真启动的第一个控制周期执行1次
if isempty(integral_val)
    integral_val = 0;
end

% ==================== 1. 控制参数（和你原PI模块参数完全一致，可直接修改）====================
Kp = 0.05;       % 比例增益，和你原设置一致
Ki = 10;         % 积分增益，和你原设置一致
Ts = 5e-5;       % 20kHz控制周期，固定不变
% ==================== 2. 物理极限设置（核心抗饱和阈值）====================
DUTY_MAX = 0.85;  % 占空比上限，避免上下管直通
DUTY_MIN = 0.15;  % 占空比下限，杜绝轻载反向电流
I_SAT_LIMIT = 4.5; % 电流传感器饱和阈值，接近±5A量程提前触发保护

% ==================== 3. 误差计算 ====================
err = I_ref - I_fb;

% ==================== 4. 比例项输出 ====================
prop_out = Kp * err;

% ==================== 5. 核心抗饱和逻辑 ====================
% 5.1 积分项预计算
integral_inc = Ki * Ts * err;
integral_pre = integral_val + integral_inc;
% 5.2 预计算不饱和的PI输出
duty_pre = prop_out + integral_pre;

% 5.3 钳位抗饱和规则：
% 仅当输出在线性区、且电流未达到传感器饱和阈值时，才允许积分累加
% 同时加入反向积分放行规则，避免积分锁死
is_duty_linear = (duty_pre < DUTY_MAX) && (duty_pre > DUTY_MIN);
is_current_unsat = (abs(I_fb) < I_SAT_LIMIT);
is_integral_allow = is_duty_linear && is_current_unsat;
is_reverse_integral = (err > 0 && integral_pre < 0) || (err < 0 && integral_pre > 0);

if is_integral_allow || is_reverse_integral
    integral_val = integral_pre;
end

% ==================== 6. 最终占空比计算 + 硬限幅兜底 ====================
duty_out = prop_out + integral_val;
duty_out = min(max(duty_out, DUTY_MIN), DUTY_MAX);

== matlab function single_phase_grid_inverter/rc滤波1 ==
  data: u input; y output
function y = fcn(u)
% 一阶RC低通滤波（数字等效实现）
% 适配：仿真步长 Ts=1e-6s（Fs=1MHz），截止频率 fc=4.7kHz
% 输入：u - 原始信号
% 输出：y - RC滤波后的信号

% persistent 变量保存上一时刻的输出（RC滤波的状态）
persistent y_prev;

% ---------------- 固定参数（已按你的需求预计算） ----------------
fc = 4700;   % 截止频率：4.7kHz
Ts = 1e-6;   % 仿真步长：1us（1e-6s）
tau = 1/(2*pi*fc); % RC时间常数 τ=RC=1/(2πfc)
alpha = exp(-Ts/tau); % 滤波系数（RC离散化核心）
% ----------------------------------------------------------------

% 初始化状态（仅第一次调用时执行，默认初始输出为0）
if isempty(y_prev)
    y_prev = 0;
end

% 一阶RC低通的离散差分方程（和真实RC电路特性完全等效）
y = alpha * y_prev + (1 - alpha) * u;

% 更新状态，为下一个仿真步准备
y_prev = y;

end

== matlab function single_phase_grid_inverter/rc滤波2 ==
  data: u input; y output
function y = fcn(u)
% 一阶RC低通滤波（数字等效实现）
% 适配：仿真步长 Ts=1e-6s（Fs=1MHz），截止频率 fc=4.7kHz
% 输入：u - 原始信号
% 输出：y - RC滤波后的信号

% persistent 变量保存上一时刻的输出（RC滤波的状态）
persistent y_prev;

% ---------------- 固定参数（已按你的需求预计算） ----------------
fc = 4700;   % 截止频率：4.7kHz
Ts = 1e-6;   % 仿真步长：1us（1e-6s）
tau = 1/(2*pi*fc); % RC时间常数 τ=RC=1/(2πfc)
alpha = exp(-Ts/tau); % 滤波系数（RC离散化核心）
% ----------------------------------------------------------------

% 初始化状态（仅第一次调用时执行，默认初始输出为0）
if isempty(y_prev)
    y_prev = 0;
end

% 一阶RC低通的离散差分方程（和真实RC电路特性完全等效）
y = alpha * y_prev + (1 - alpha) * u;

% 更新状态，为下一个仿真步准备
y_prev = y;

end

== matlab function single_phase_grid_inverter/1.5倍延时 ==
  data: u input; y output
function y = SecondOrderPadeDelay_1p5Ts(u)
% 二阶Padé逼近1.5Ts延迟模块（直接从闭环仿真提取，已验证直流增益=1）
% 输入：u - 待延迟的信号（如PR控制器输出）
% 输出：y - 延迟后的信号
% 适配：与你的闭环仿真参数100%匹配，直流增益严格等于1

persistent u_prev1 u_prev2 y_prev1 y_prev2 first_run

%% 初始化：仅首次运行
if isempty(first_run)
    % 初始化状态变量（二阶需要2个历史输入+2个历史输出）
    u_prev1 = 0;
    u_prev2 = 0;
    y_prev1 = 0;
    y_prev2 = 0;
    
    first_run = true;
end

%% 【核心】直接从闭环仿真提取的系数（已验证直流增益=1）
b0 = 0.076923076923077;
b1 = 0.153846153846154;
b2 = 1.000000000000000;
a1 = -0.153846153846154;
a2 = -0.076923076923077;

%% 二阶离散差分方程计算延迟输出
y = b0*u + b1*u_prev1 + b2*u_prev2 ...
    + a1*y_prev1 + a2*y_prev2;

%% 更新状态变量（供下一时刻使用）
u_prev2 = u_prev1;
u_prev1 = u;
y_prev2 = y_prev1;
y_prev1 = y;
end

== matlab function single_phase_grid_inverter/rc滤波3 ==
  data: u input; y output
function y = fcn(u)
% 一阶RC低通滤波（数字等效实现）
% 适配：仿真步长 Ts=1e-6s（Fs=1MHz），截止频率 fc=4.7kHz
% 输入：u - 原始信号
% 输出：y - RC滤波后的信号

% persistent 变量保存上一时刻的输出（RC滤波的状态）
persistent y_prev;

% ---------------- 固定参数（已按你的需求预计算） ----------------
fc = 4700;   % 截止频率：4.7kHz
Ts = 1e-6;   % 仿真步长：1us（1e-6s）
tau = 1/(2*pi*fc); % RC时间常数 τ=RC=1/(2πfc)
alpha = exp(-Ts/tau); % 滤波系数（RC离散化核心）
% ----------------------------------------------------------------

% 初始化状态（仅第一次调用时执行，默认初始输出为0）
if isempty(y_prev)
    y_prev = 0;
end

% 一阶RC低通的离散差分方程（和真实RC电路特性完全等效）
y = alpha * y_prev + (1 - alpha) * u;

% 更新状态，为下一个仿真步准备
y_prev = y;

end

== matlab function single_phase_grid_inverter/MATLAB Function4 ==
  settings: updateMethod=DISCRETE
  data: u input; y output
function y = PR_Controller(u)
%#codegen
% PR控制器 + 【模仿PI的抗饱和逻辑】
% 输入 u: 误差 Iref - Ifb
% 输出 y: 调制波 ±0.9

persistent x_prev1 x_prev2 y_prev1 y_prev2 first_run ;

%% 1. PR参数
Ts = 5e-5;
Kp = 0.3;
Kr = 40.92;
w0 = 2*pi*50;
wi = pi;

%% 限幅（和你PI保持一致风格）
OUT_MAX =  0.9;
OUT_MIN = -0.9;

%% 初始化
if isempty(first_run)
    x_prev1 = 0;
    x_prev2 = 0;
    y_prev1 = 0;
    y_prev2 = 0;
    first_run = true;
end

%% 2. PR离散系数
a0_pr = 4 + 2*wi*Ts + w0^2*Ts^2;
a1_pr = 2*w0^2*Ts^2 - 8;
a2_pr = 4 - 2*wi*Ts + w0^2*Ts^2;

b0_pr = 4*Kp + 4*Kp*wi*Ts + 4*Kr*wi*Ts + Kp*w0^2*Ts^2;
b1_pr = 2*Kp*w0^2*Ts^2 - 8*Kp;
b2_pr = 4*Kp - 4*Kp*wi*Ts - 4*Kr*wi*Ts + Kp*w0^2*Ts^2;

%% 3. 计算未限幅输出
y_unlim = (b0_pr*u + b1_pr*x_prev1 + b2_pr*x_prev2 ...
    - a1_pr*y_prev1 - a2_pr*y_prev2) / a0_pr;

%% ===================== 【完全模仿你PI的抗饱和逻辑】 =====================
duty_pre = y_unlim;

% 1. 判断是否在线性区
is_linear = (duty_pre < OUT_MAX) && (duty_pre > OUT_MIN);

% 2. 反向积分判断（让积分能退出来，不锁死）
is_reverse = (u > 0 && duty_pre < 0) || (u < 0 && duty_pre > 0);

% 3. 只有 线性区 或 反向退饱和 时，才更新状态
if is_linear || is_reverse
    % 更新状态
    x_prev2 = x_prev1;
    x_prev1 = u;
    y_prev2 = y_prev1;
    y_prev1 = y_unlim;
end

%% ===================== 最终限幅 =====================
y = max(min(y_unlim, OUT_MAX), OUT_MIN);

end

== matlab function single_phase_grid_inverter/rc滤波4 ==
  data: u input; y output
function y = fcn(u)
% 一阶RC低通滤波（数字等效实现）
% 适配：仿真步长 Ts=1e-6s（Fs=1MHz），截止频率 fc=4.7kHz
% 输入：u - 原始信号
% 输出：y - RC滤波后的信号

% persistent 变量保存上一时刻的输出（RC滤波的状态）
persistent y_prev;

% ---------------- 固定参数（已按你的需求预计算） ----------------
fc = 4700;   % 截止频率：4.7kHz
Ts = 1e-6;   % 仿真步长：1us（1e-6s）
tau = 1/(2*pi*fc); % RC时间常数 τ=RC=1/(2πfc)
alpha = exp(-Ts/tau); % 滤波系数（RC离散化核心）
% ----------------------------------------------------------------

% 初始化状态（仅第一次调用时执行，默认初始输出为0）
if isempty(y_prev)
    y_prev = 0;
end

% 一阶RC低通的离散差分方程（和真实RC电路特性完全等效）
y = alpha * y_prev + (1 - alpha) * u;

% 更新状态，为下一个仿真步准备
y_prev = y;

end

== matlab function single_phase_grid_inverter/MATLAB Function3 ==
  data: ua input; VT1 output; uanot input; ub input; ubnot input; t input; VT2 output; VT3 output; VT4 output
function [VT1, VT2, VT3, VT4] = fcn(ua, uanot, ub, ubnot, t)
% 分段 PWM 输出控制
% t < 0.25s       → 全 0
% 0.25s ≤ t < 1s  → 正常输出
% t ≥ 1s          → 再次全 0

if t < 0.25
    % 第一段：小于0.25秒 → 全关
    VT1 = 0.0;
    VT2 = 0.0;
    VT3 = 0.0;
    VT4 = 0.0;
elseif t < 0.9
    % 第二段：0.25~1秒 → 正常输出
    VT1 = double(ua);
    VT2 = double(uanot);
    VT3 = double(ub);
    VT4 = double(ubnot);
else
    % 第三段：大于等于1秒 → 再次全关
    VT1 = 0.0;
    VT2 = 0.0;
    VT3 = 0.0;
    VT4 = 0.0;
end
